simulink model "bus_outputAsBusComplex"  (Simulink 8.0)
settings: Solver=ode45  StartTime=0.0  StopTime=10.0  RelTol=1e-3
settings Model: Creator=massif  LastModifiedBy=massif

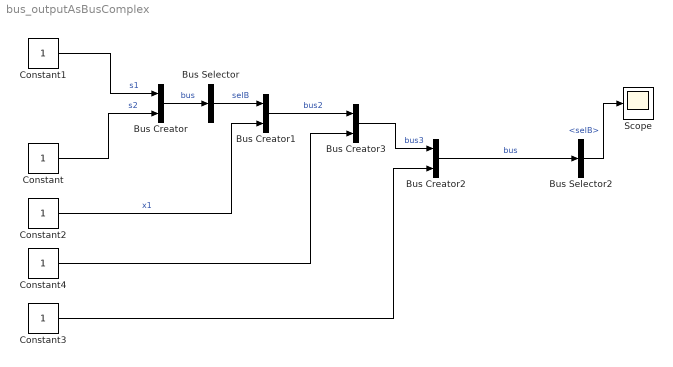
== system bus_outputAsBusComplex ==
  Bus Creator{,1..3} (4 alike) : BusCreator  Inputs=2
  Bus Selector : BusSelector  OutputSignals=s1,s2  OutputAsBus=on
  Bus Selector2 : BusSelector  OutputSignals=bus3.bus2.selB
  Constant{,1..4} (5 alike) : Constant
  Scope : Scope
  wires:
  Constant1/1 -> Bus Creator/1  "s1"
  Bus Creator/1 -> Bus Selector/1  "bus"
  Bus Selector/1 -> Bus Creator1/1  "selB"
  Constant/1 -> Bus Creator/2  "s2"
  Bus Creator3/1 -> Bus Creator2/1  "bus3"
  Constant2/1 -> Bus Creator1/2  "x1"
  Bus Creator1/1 -> Bus Creator3/1  "bus2"
  Constant3/1 -> Bus Creator2/2
  Bus Creator2/1 -> Bus Selector2/1  "bus"
  Bus Selector2/1 -> Scope/1  "<selB>"
  Constant4/1 -> Bus Creator3/2
